simulink model "hw6_linear"  (R2024a)
settings: Solver=VariableStepAuto  StartTime=0.0  StopTime=10.0  RelTol=1e-3
values from neighbouring files (symbols this model uses):
  u_bar = 1.89    [hw6main.m]
  y = 8    [hw6main.m]
  y_bar = 4    [hw6main.m]
settings Model: Creator=xinchen  LastModifiedBy=xinchen

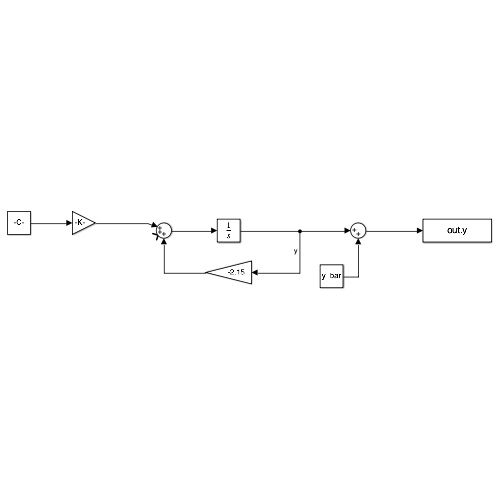
[thumbnail: Simulink's stored preview of the top-level diagram]
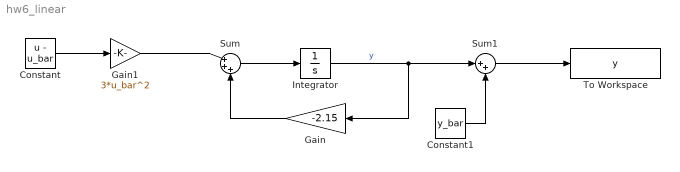
== system hw6_linear ==
  Constant : Constant  Value=u - u_bar
  Constant1 : Constant  Value=y_bar
  Gain : Gain  Gain=-2.15
  Gain1 : Gain  Gain=3*u_bar^2
  Integrator : Integrator  InitialCondition=y - y_bar
  Sum : Sum  Inputs=|+++
  Sum1 : Sum  Inputs=|++
  To Workspace : ToWorkspace  VariableName=y  SampleTime=-1
  wires:
  Constant/1 -> Gain1/1
  Integrator/1 -> Sum1/1, Gain/1  "y"
  Sum/1 -> Integrator/1
  Gain/1 -> Sum/3
  Gain1/1 -> Sum/1
  Sum1/1 -> To Workspace/1
  Constant1/1 -> Sum1/2
